simulink model "sim_rbf"  (R2023a)
settings: Solver=VariableStepAuto  StartTime=0.0  StopTime=10.0  RelTol=1e-3
settings Model: Creator=mluser  LastModifiedBy=mluser

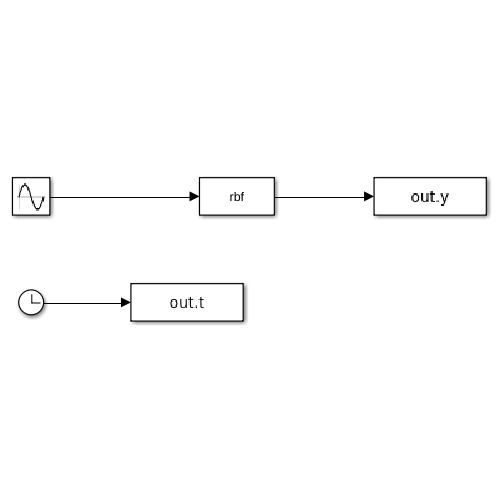
[thumbnail: Simulink's stored preview of the top-level diagram]
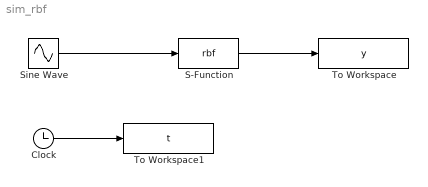
== system sim_rbf ==
  Clock : Clock
      settings: Decimation=30
  S-Function : S-Function  FunctionName=rbf  SFunctionDeploymentMode=off  EnableBusSupport=off
  Sine Wave : Sin  SampleTime=0
  To Workspace : ToWorkspace  VariableName=y  SampleTime=-1
  To Workspace1 : ToWorkspace  VariableName=t  SampleTime=-1
  wires:
  Sine Wave/1 -> S-Function/1
  S-Function/1 -> To Workspace/1
  Clock/1 -> To Workspace1/1
